simulink model "TankFilling"  (R2020b)
settings: Solver=VariableStepAuto  StartTime=0.0  StopTime=10  RelTol=1e-3
values from neighbouring files (symbols this model uses):
  a_in = 1    [TankFillingScript.m]
  c = 16    [TankFillingScript.m]
  Q_in = 1    [TankFillingScript.m]
settings Model: Creator=StevensUser  LastModifiedBy=mreiff

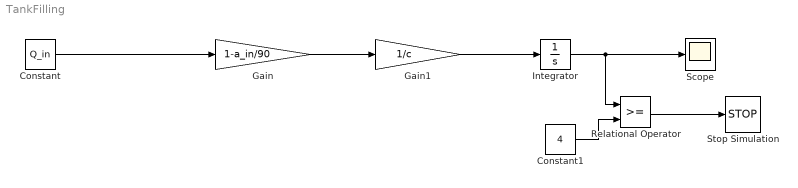
== system TankFilling ==
  Constant : Constant  Value=Q_in
  Constant1 : Constant  Value=4
  Gain : Gain  Gain=1-a_in/90
  Gain1 : Gain  Gain=1/c
  Integrator : Integrator
  Relational Operator : RelationalOperator  OutDataTypeStr=boolean  RndMeth=Simplest
  Scope : Scope
  Stop Simulation : Stop
  wires:
  Constant/1 -> Gain/1
  Gain/1 -> Gain1/1
  Gain1/1 -> Integrator/1
  Relational Operator/1 -> Stop Simulation/1
  Constant1/1 -> Relational Operator/2
  Integrator/1 -> Relational Operator/1, Scope/1
